simulink model "sldemo_mdlref_fcncall_cntr"  (Simulink 7.6)
settings: Solver=FixedStepDiscrete  StartTime=0.0  StopTime=10.0  FixedStep=1  MaxStep=inf  RelTol=1e-3  SampleTimeConstraint=STIndependent
Description:
  | Function-Call Counter
  | 
  | Illustration of a function-call model of a triggered counter. The
  | counter bounds are provided through the input ports of the model.
  | The counter increments each time the model is triggered.
  | 
  | During simulation, a function-call model is implicitly triggered by the
  | solver.  Using a fixed-step solver configures the model to simulate
  | using evenly spaced time steps. Using a variable-step solver allows
  | the model to simulate using unevenly spaced time steps.
settings Model: Creator=The MathWorks Inc.  ExtModeAutoUpdateStatusClock=off
settings DataIOCC: ExternalInput=[0 10 0; 10 10 0]  LoadExternalInput=on  SaveFormat=StructureWithTime  SignalLoggingName=logsOut  OutputOption=AdditionalOutputTimes  OutputTimes=[0,1,9,10]
settings OptimizationCC: InlineParams=on  InlineInvariantSignals=on  InitFltsAndDblsToZero=on
settings DebuggingCC: SaveWithParameterizedLinksMsg=none  CheckExecutionContextPreStartOutputMsg=on  CheckExecutionContextRuntimeOutputMsg=on  SolverPrmCheckMsg=none  MultiTaskDSMMsg=warning  MultiTaskCondExecSysMsg=none  SigSpecEnsureSampleTimeMsg=none  StrictBusMsg=ErrorOnBusTreatedAsVector
settings HardwareCC: TargetHWDeviceType=32-bit Generic
settings ModelReferenceCC: UpdateModelReferenceTargets=IfOutOfDate  CheckModelReferenceTargetMessage=none
settings RTWCC: GenerateReport=on  ProcessScript=grt_make_rtw_hook  LaunchReport=on  IncludeERTFirstTime=on
settings CodeAppCC: MaxIdLength=100
settings GRTTargetCC: TargetFcnLib=ansi_tfl_tmw.mat

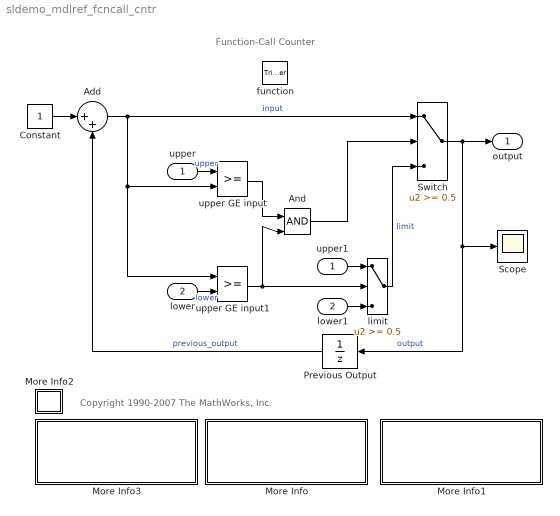
== system sldemo_mdlref_fcncall_cntr ==
  note: Copyright 1990-2007 The MathWorks, Inc.
  note: Function-Call Counter
  upper : Inport
  lower : Inport  Port=2
  function : TriggerPort  TriggerType=function-call  SampleTime=0.5
  " limit" : Switch  Threshold=0.5  SaturateOnIntegerOverflow=on  InputSameDT=on
  Add : Sum  Inputs=|++
  And : Logic  IconShape=distinctive
      settings: AttributesFormatString=%<Operator>
  Constant : Constant
  More Info : Subsystem
      settings: OpenFcn=|
      | set_param(bdroot(gcb),'Solver','FixedStepDiscrete');
      | set_param(bdroot(gcb),'SampleTimeConstraint', 'Unconstrained');
      | set_param(bdroot(gcb),'FixedStep','1');
      | set_param(bdroot(gcb),'SolverMode','Auto');
      mask Display: disp('Fixed-step solver\nTs=1\n(double-click)');
  More Info1 : Subsystem
      settings: OpenFcn=|
      | set_param(bdroot(gcb),'Solver','VariableStepDiscrete');
      | set_param(bdroot(gcb),'MaxStep','inf');
      | set_param(bdroot(gcb),'OutputOption','AdditionalOutputTimes');
      | set_param(bdroot(gcb),'OutputTimes','[0,1,9,10]');
      mask Display: disp('Variable-step solver\n T=[0,1,9,10]\n(double-click)');
  More Info2 : Subsystem
      settings: OpenFcn=showdemo(bdroot(gcs))
      mask Display: disp('?')
  More Info3 : Subsystem
      settings: OpenFcn=|
      | set_param(bdroot(gcb),'Solver','FixedStepDiscrete');
      | set_param(bdroot(gcb),'SampleTimeConstraint','STIndependent');
      mask Display: disp('Fixed-step solver\nSample-Time Independent\n(double-click)');
  Previous Output : UnitDelay  SampleTime=-1
  Scope : Scope
      settings: TimeRange=10  YMin=0  YMax=10
  Switch : Switch  Threshold=0.5  SaturateOnIntegerOverflow=on  InputSameDT=on
  lower1 : InportShadow  Port=2
  upper GE input : RelationalOperator  Priority=0  InputSameDT=on
      settings: AttributesFormatString=\n
  upper GE input1 : RelationalOperator  Priority=0  InputSameDT=on
      settings: AttributesFormatString=\n
  upper1 : InportShadow  Port=1
  output : Outport
  wires:
  Switch/1 -> output/1, Previous Output/1, Scope/1  "output"
  " limit"/1 -> Switch/3  "limit"
  upper GE input/1 -> And/1
  Previous Output/1 -> Add/2  "previous_output"
  upper/1 -> upper GE input/1  "upper"
  upper GE input1/1 -> And/2, " limit"/2
  And/1 -> Switch/2
  Add/1 -> Switch/1, upper GE input/2, upper GE input1/1  "input"
  Constant/1 -> Add/1
  lower/1 -> upper GE input1/2  "lower"
  upper1/1 -> " limit"/1
  lower1/1 -> " limit"/3

== system sldemo_mdlref_fcncall_cntr/More Info ==

== system sldemo_mdlref_fcncall_cntr/More Info1 ==

== system sldemo_mdlref_fcncall_cntr/More Info2 ==

== system sldemo_mdlref_fcncall_cntr/More Info3 ==
